simulink model "inc_enc_v26"  (R2022b)
settings: Solver=FixedStepDiscrete  StartTime=0.0  StopTime=SimulationsDauer  RelTol=1e-3
values from neighbouring files (symbols this model uses):
  f_ISR = 40e3    (= 40000)    [Init_IncreEncoder_v26.m]
  IncPerTurn = 2500    [Init_IncreEncoder_v26.m]
  inital_zero_speed_timeout = speed_timeout_in_s*f_fpga    (= 5000)    [Init_IncreEncoder_v26.m]
  n_max = 6000    [Init_IncreEncoder_v26.m]
  Offset_Position_elec = 42    [Init_IncreEncoder_v26.m]
  Offset_Position_mech = 753    [Init_IncreEncoder_v26.m]
  OmegaPerOverSampl = 1500*((2*pi)/60)    (= 157.079632679)    [Init_IncreEncoder_v26.m]
  Periode = abs(1/Striche_pro_Sekunde)    [Init_IncreEncoder_v26.m]
  Phase_Delay_A = Periode/8    [Init_IncreEncoder_v26.m]
  Phase_Delay_B = -Periode/8    [Init_IncreEncoder_v26.m]
  PolePair = 10    [Init_IncreEncoder_v26.m]
  QuadratureFactor = 4    [Init_IncreEncoder_v26.m]
  reciprocal_iterations = 3    [Init_IncreEncoder_v26.m]
  T_fpga = 1/f_fpga    (= 1e-08)    [Init_IncreEncoder_v26.m]
  T_mech = 1e-08    [Init_IncreEncoder_v26.m]
undefined symbols (not defined in the file or in its folder): CW_CCW_Switch, d_axis_hit_CompareValue, DiscIntNeverNeededParam
libraries: hdlsllib x4, dspsrcs4 x3, dspswit3 x2, spsEdgeDetectorLib x2, simulink_extras x1
(part 1 of 2)
settings Model: DataTypeOverride=Off  Creator=Wendel_ELSYS  LastModifiedBy=Admin
settings SolverCC: ConcurrentTasks=on  AlgebraicLoopSolver=TrustRegion  MinimalZcImpactIntegration=on
settings DataIOCC: LimitDataPoints=on  SaveFormat=Array
settings OptimizationCC: BlockReduction=off  ConditionallyExecuteInputs=off  DefaultParameterBehavior=Inlined  InheritOutputTypeSmallerThanSingle=on  LifeSpan=inf
settings DebuggingCC: ReadBeforeWriteMsg=DisableAll  WriteAfterWriteMsg=DisableAll  WriteAfterReadMsg=DisableAll  AlgebraicLoopMsg=error  SingleTaskRateTransMsg=error  ParameterOverflowMsg=none  UnconnectedInputMsg=warning  UnconnectedOutputMsg=warning  UnconnectedLineMsg=warning  SFUnexpectedBacktrackingDiag=warning  SFNoUnconditionalDefaultTransitionDiag=warning  SFExecutionAtInitializationDiag=none  SFMachineParentedDataDiag=warning  ArithmeticOperatorsInVariantConditions=warning
settings HardwareCC: ProdBitPerPointer=32  ProdBitPerSizeT=32  ProdBitPerPtrDiffT=32  ProdLargestAtomicFloat=None  ProdIntDivRoundTo=Undefined  ProdEndianess=Unspecified  ProdWordSize=32  ProdHWDeviceType=ASIC/FPGA->ASIC/FPGA  ProdEqTarget=off
settings ModelReferenceCC: UpdateModelReferenceTargets=IfOutOfDate  EnableRefExpFcnMdlSchedulingChecks=on  PropagateSignalLabelsOutOfModel=off
settings SFSimCC: SFSimEcho=off  SimUseLocalCustomCode=off  CustomCodeUndefinedFunction=UseInterfaceOnly
settings RTWCC: RTWUseLocalCustomCode=off  DLArmComputeVersion=19.05
settings CodeAppCC: StateflowObjectComments=on
settings GRTTargetCC: TargetLangStandard=C89/C90 (ANSI)
settings ConfigComp: CovMetricSettings=dw  CovSaveCumulativeToWorkspaceVar=on  CovSaveSingleToWorkspaceVar=on  CovExternalEMLEnable=off
settings SimscapeCC: SimscapeNormalizeSystem=off

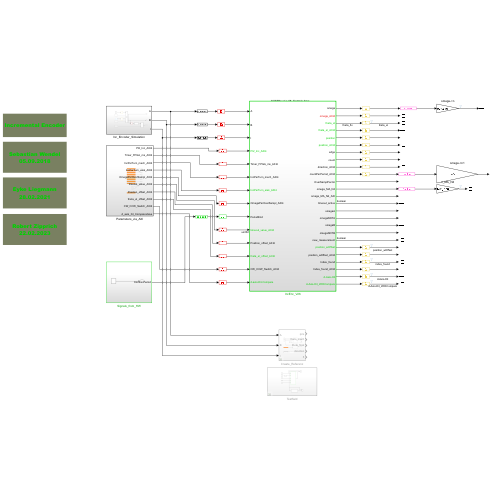
[thumbnail: Simulink's stored preview of the top-level diagram]
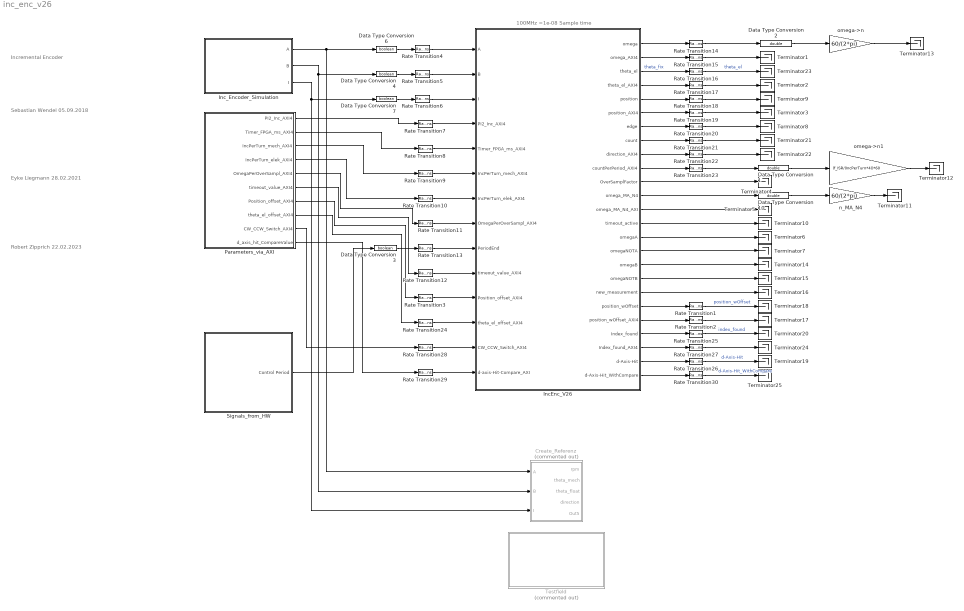
== system inc_enc_v26 ==
  note: 100MHz =1e-08 Sample time
  note: Sebastian Wendel
      | 05.09.2018
  note: Incremental Encoder
  note: Eyke Liegmann
      | 28.02.2021
  note: Robert Zipprich
      | 22.02.2023
  Create_Referenz : Subsystem  Commented=on
  Data Type Conversion1 : DataTypeConversion  OutDataTypeStr=double  SaturateOnIntegerOverflow=off  RndMeth=Floor
  Data Type Conversion10 : DataTypeConversion  OutDataTypeStr=double  SaturateOnIntegerOverflow=off  RndMeth=Floor
  Data Type Conversion2 : DataTypeConversion  OutDataTypeStr=double  SaturateOnIntegerOverflow=off  RndMeth=Floor
  Data Type Conversion{3..4,6..7} (4 alike) : DataTypeConversion  OutDataTypeStr=boolean  SaturateOnIntegerOverflow=off  RndMeth=Floor
  IncEnc_V26 : Subsystem  TreatAsAtomicUnit=on
  Inc_Encoder_Simulation : Subsystem
  Parameters_via_AXI : Subsystem
  Rate Transition{1..2,14..23,25..27,30} (16 alike) : RateTransition  Deterministic=off  OutPortSampleTime=T_mech
  Rate Transition{3..13,24,28..29} (14 alike) : RateTransition  Deterministic=off  OutPortSampleTime=T_fpga
  Signals_from_HW : Subsystem
  Terminator{1..25} (25 alike) : Terminator
  Testfield : Subsystem  Commented=on
  n_MA_N4 : Gain  Gain=60/(2*pi)  OutDataTypeStr=double
  omega->n : Gain  Gain=60/(2*pi)  OutDataTypeStr=double
  omega->n1 : Gain  Gain=(f_ISR/(IncPerTurn*4))*60  OutDataTypeStr=double
  wires:
  Data Type Conversion6/1 -> Rate Transition4/1
  Data Type Conversion4/1 -> Rate Transition5/1
  Data Type Conversion7/1 -> Rate Transition6/1
  IncEnc_V26/1(omega) -> Rate Transition14/1
  IncEnc_V26/9(direction_AXI4) -> Rate Transition22/1
  IncEnc_V26/7(edge) -> Rate Transition20/1
  IncEnc_V26/8(count) -> Rate Transition21/1
  IncEnc_V26/3(theta_el) -> Rate Transition16/1  "theta_fix"
  IncEnc_V26/5(position) -> Rate Transition18/1
  IncEnc_V26/4(theta_el_AXI4) -> Rate Transition17/1
  IncEnc_V26/2(omega_AXI4) -> Rate Transition15/1
  omega->n/1 -> Terminator13/1
  Data Type Conversion2/1 -> omega->n/1
  Data Type Conversion1/1 -> omega->n1/1
  IncEnc_V26/10(countPerPeriod_AXI4) -> Rate Transition23/1
  Data Type Conversion3/1 -> Rate Transition13/1
  IncEnc_V26/6(position_AXI4) -> Rate Transition19/1
  Rate Transition4/1 -> IncEnc_V26/1(A)
  Rate Transition5/1 -> IncEnc_V26/2(B)
  Rate Transition6/1 -> IncEnc_V26/3(I)
  Rate Transition7/1 -> IncEnc_V26/4(PI2_Inc_AXI4)
  Rate Transition8/1 -> IncEnc_V26/5(Timer_FPGA_ms_AXI4)
  Rate Transition9/1 -> IncEnc_V26/6(IncPerTurn_mech_AXI4)
  Rate Transition10/1 -> IncEnc_V26/7(IncPerTurn_elek_AXI4)
  Rate Transition11/1 -> IncEnc_V26/8(OmegaPerOverSampl_AXI4)
  Rate Transition13/1 -> IncEnc_V26/9(PeriodEnd)
  Rate Transition14/1 -> Data Type Conversion2/1
  Rate Transition15/1 -> Terminator1/1
  Rate Transition17/1 -> Terminator2/1
  Rate Transition19/1 -> Terminator3/1
  Rate Transition23/1 -> Data Type Conversion1/1
  IncEnc_V26/11(OverSamplFactor) -> Terminator4/1
  IncEnc_V26/12(omega_MA_N4) -> Data Type Conversion10/1
  IncEnc_V26/13(omega_MA_N4_AXI) -> Terminator5/1
  Data Type Conversion10/1 -> n_MA_N4/1
  Rate Transition12/1 -> IncEnc_V26/10(timeout_value_AXI4)
  IncEnc_V26/14(timeout_active) -> Terminator10/1
  Rate Transition20/1 -> Terminator8/1
  Rate Transition18/1 -> Terminator9/1
  n_MA_N4/1 -> Terminator11/1
  omega->n1/1 -> Terminator12/1
  IncEnc_V26/15(omegaA) -> Terminator6/1
  IncEnc_V26/18(omegaNOTB) -> Terminator15/1
  IncEnc_V26/17(omegaB) -> Terminator14/1
  IncEnc_V26/16(omegaNOTA) -> Terminator7/1
  IncEnc_V26/19(new_measurement) -> Terminator16/1
  Parameters_via_AXI/1(PI2_Inc_AXI4) -> Rate Transition7/1
  Parameters_via_AXI/2(Timer_FPGA_ms_AXI4) -> Rate Transition8/1
  Parameters_via_AXI/3(IncPerTurn_mech_AXI4) -> Rate Transition9/1
  Parameters_via_AXI/4(IncPerTurn_elek_AXI4) -> Rate Transition10/1
  Parameters_via_AXI/5(OmegaPerOverSampl_AXI4) -> Rate Transition11/1
  Parameters_via_AXI/6(timeout_value_AXI4) -> Rate Transition12/1
  Inc_Encoder_Simulation/2(B) -> Create_Referenz/2(B), Data Type Conversion4/1
  Inc_Encoder_Simulation/3(I) -> Create_Referenz/3(I), Data Type Conversion7/1
  Inc_Encoder_Simulation/1(A) -> Data Type Conversion6/1, Create_Referenz/1(A)
  Signals_from_HW/1(Control Period) -> Data Type Conversion3/1
  Rate Transition1/1 -> Terminator18/1  "position_wOffset"
  Rate Transition2/1 -> Terminator17/1
  IncEnc_V26/21(position_wOffset_AXI4) -> Rate Transition2/1
  IncEnc_V26/20(position_wOffset) -> Rate Transition1/1
  Rate Transition3/1 -> IncEnc_V26/11(Position_offset_AXI4)
  Parameters_via_AXI/7(Position_offset_AXI4) -> Rate Transition3/1
  Rate Transition24/1 -> IncEnc_V26/12(theta_el_offset_AXI4)
  Parameters_via_AXI/8(theta_el_offset_AXI4) -> Rate Transition24/1
  IncEnc_V26/22(Index_found) -> Rate Transition25/1
  Rate Transition25/1 -> Terminator20/1  "index_found"
  Rate Transition26/1 -> Terminator19/1  "d-Axis-Hit"
  IncEnc_V26/24(d-Axis-Hit) -> Rate Transition26/1
  Rate Transition22/1 -> Terminator22/1
  Rate Transition21/1 -> Terminator21/1
  Rate Transition16/1 -> Terminator23/1  "theta_el"
  Rate Transition27/1 -> Terminator24/1
  IncEnc_V26/23(Index_found_AXI4) -> Rate Transition27/1
  Rate Transition28/1 -> IncEnc_V26/13(CW_CCW_Switch_AXI4)
  Parameters_via_AXI/9(CW_CCW_Switch_AXI4) -> Rate Transition28/1
  Rate Transition29/1 -> IncEnc_V26/14(d-axis-Hit-Compare_AXI)
  Parameters_via_AXI/10(d_axis_hit_CompareValue) -> Rate Transition29/1
  IncEnc_V26/25(d-Axis-Hit_WithCompare) -> Rate Transition30/1
  Rate Transition30/1 -> Terminator25/1  "d-Axis-Hit_WithCompare"

== system inc_enc_v26/Create_Referenz ==
  note: Überprüfen der Ausgabe:
      | (1/((Wert in Periodfelt von Counter)*Inkremente))*60
      | z.B. (1/((2.5*0.000001)*5000))*60
  A : Inport
  B : Inport  Port=2
  I : Inport  Port=3
  HardwareTimer_FPGA_in_ms*InCrements1 : Constant  Value=T_mech*IncPerTurn  OutDataTypeStr=double  SampleTime=T_mech
  IncrementalEncoder_Floating : Subsystem  Commented=on
  "daQuadraturEncoder " : Gain  Commented=on  Gain=4
  n_aus_theta : Subsystem  Commented=on  TreatAsAtomicUnit=on
  poles : Constant  Value=PolePair  OutDataTypeStr=uint8  SampleTime=T_mech
  rpm : Outport
  theta_mech : Outport  Port=2
  theta_float : Outport  Port=3
  direction : Outport  Port=4
  Out5 : Outport  Port=5
  wires:
  n_aus_theta/1(rpm) -> "daQuadraturEncoder "/1
  A/1 -> IncrementalEncoder_Floating/1(A), n_aus_theta/1(count)
  B/1 -> IncrementalEncoder_Floating/2(B)
  IncrementalEncoder_Floating/3(theta_elec) -> theta_float/1  "theta_float"
  poles/1 -> IncrementalEncoder_Floating/4(poles)
  I/1 -> IncrementalEncoder_Floating/3(I)
  HardwareTimer_FPGA_in_ms*InCrements1/1 -> n_aus_theta/2(T)
  IncrementalEncoder_Floating/4(direction) -> direction/1
  IncrementalEncoder_Floating/1(rpm) -> rpm/1
  "daQuadraturEncoder "/1 -> Out5/1
  IncrementalEncoder_Floating/2(theta_mech) -> theta_mech/1

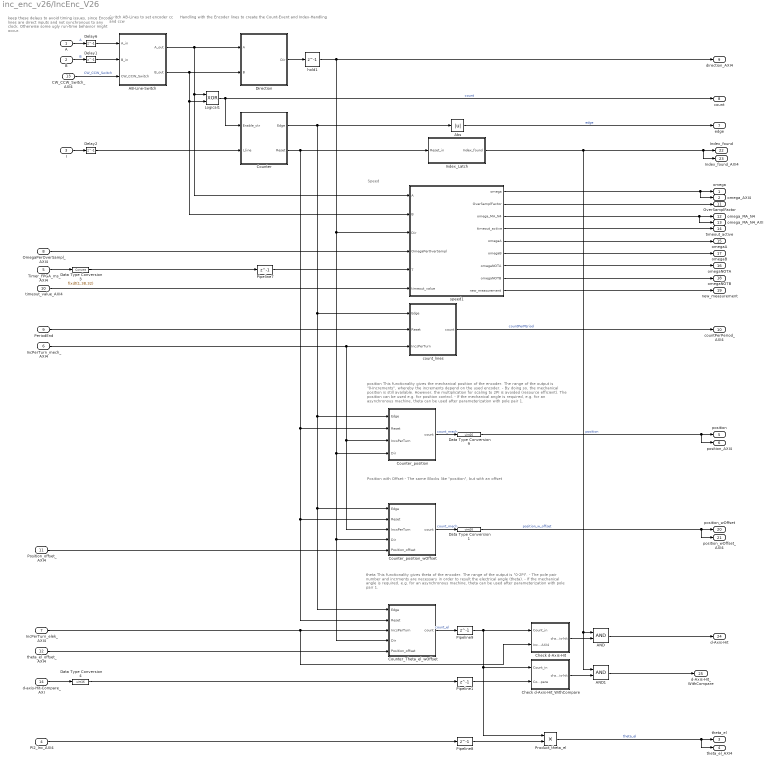
== system inc_enc_v26/IncEnc_V26 ==
  note: Switch AB-Lines to set
      | encoder cc and ccw
  note: Handling with the Encoder lines to create the Count-Event and Index-Handling
  note: Speed
  note: position
      | This functionality gives the mechanical position of the encoder. The range of the output is "0-Increments", whereby the increments depend on the used encoder.
      | - By doing so, the mechanical position is still available. However, the multiplication for scaling to 2PI is avoided (resource efficient). The position can be used e.g. for position control.
      | - If the mechanical angle is required, e.g. for an asynchronous machine, theta can be used after parameterization with pole pair 1.
  note: theta
      | This functionality gives theta of the encoder. The range of the output is "0-2PI".
      | - The pole pair number and incrments are necessary in order to result the electrical angle (theta).
      | - If the mechanical angle is required, e.g. for an asynchronous machine, theta can be used after parameterization with pole pair 1.
  note: keep these delays to avoid timing issues,
      | since Encoder lines are direct inputs and
      | not synchronous to any clock.
      | Otherwise some ugly run-time
      | behavior might occur.
  note: Position with Offset
      | - The same Blocks like "position", but with an offset
  A : Inport
  B : Inport  Port=2
  I : Inport  Port=3
  PI2_Inc_AXI4 : Inport  Port=4
  Timer_FPGA_ms_AXI4 : Inport  Port=5
  IncPerTurn_mech_AXI4 : Inport  Port=6
  IncPerTurn_elek_AXI4 : Inport  Port=7
  OmegaPerOverSampl_AXI4 : Inport  Port=8
  PeriodEnd : Inport  Port=9
  timeout_value_AXI4 : Inport  Port=10  OutDataTypeStr=uint32
  Position_offset_AXI4 : Inport  Port=11
  theta_el_offset_AXI4 : Inport  Port=12
  CW_CCW_Switch_AXI4 : Inport  Port=13
  d-axis-Hit-Compare_AXI : Inport  Port=14
  AB-Line-Switch : Subsystem
  AND : Logic  AllPortsSameDT=off  OutDataTypeStr=boolean
  AND1 : Logic  AllPortsSameDT=off  OutDataTypeStr=boolean
  Abs : Abs  OutDataTypeStr=fixdt(0,1,0)  RndMeth=Simplest  SaturateOnIntegerOverflow=off
  Check d-Axis-Hit : Subsystem
  Check d-Axis-Hit_WithCompare : Subsystem
  Counter : Subsystem  TreatAsAtomicUnit=on
  Counter_Theta_el_wOffset : Subsystem  TreatAsAtomicUnit=on
  Counter_position : Subsystem  TreatAsAtomicUnit=on
  Counter_position_wOffset : Subsystem  TreatAsAtomicUnit=on
  Data Type Conversion1 : DataTypeConversion  OutDataTypeStr=uint16  SaturateOnIntegerOverflow=off  RndMeth=Floor
  Data Type Conversion3 : DataTypeConversion  OutDataTypeStr=fixdt(1,38,32)  SaturateOnIntegerOverflow=off  RndMeth=Floor
  Data Type Conversion4 : DataTypeConversion  OutDataTypeStr=uint16  SaturateOnIntegerOverflow=off  RndMeth=Floor
  Data Type Conversion9 : DataTypeConversion  OutDataTypeStr=uint16  SaturateOnIntegerOverflow=off  RndMeth=Floor
  Delay1 : Delay  DelayLength=1  InitialCondition=0
  Delay2 : Delay  DelayLength=1  InitialCondition=0
  Delay6 : Delay  DelayLength=1  InitialCondition=0
  Direction : Subsystem  TreatAsAtomicUnit=on
  Index_Latch : Subsystem
  Logical1 : Logic  Operator=XOR  AllPortsSameDT=off  OutDataTypeStr=boolean
  Pipeline{1,7..9} (4 alike) : Delay  DelayLength=1
  Product_theta_el : Product  OutMin=[0]  OutMax=[2*pi]  OutDataTypeStr=fixdt(1,24,20)
  count_lines : Subsystem  TreatAsAtomicUnit=on
  hold1 : Delay  DelayLength=1
  speed1 : Subsystem
  omega : Outport  VectorParamsAs1DForOutWhenUnconnected=off
  omega_AXI4 : Outport  Port=2  VectorParamsAs1DForOutWhenUnconnected=off
  theta_el : Outport  Port=3  VectorParamsAs1DForOutWhenUnconnected=off
  theta_el_AXI4 : Outport  Port=4  VectorParamsAs1DForOutWhenUnconnected=off
  position : Outport  Port=5  VectorParamsAs1DForOutWhenUnconnected=off
  position_AXI4 : Outport  Port=6  VectorParamsAs1DForOutWhenUnconnected=off
  edge : Outport  Port=7  VectorParamsAs1DForOutWhenUnconnected=off
  count : Outport  Port=8  VectorParamsAs1DForOutWhenUnconnected=off
  direction_AXI4 : Outport  Port=9  VectorParamsAs1DForOutWhenUnconnected=off
  countPerPeriod_AXI4 : Outport  Port=10  VectorParamsAs1DForOutWhenUnconnected=off
  OverSamplFactor : Outport  Port=11  VectorParamsAs1DForOutWhenUnconnected=off
  omega_MA_N4 : Outport  Port=12  VectorParamsAs1DForOutWhenUnconnected=off
  omega_MA_N4_AXI : Outport  Port=13  VectorParamsAs1DForOutWhenUnconnected=off
  timeout_active : Outport  Port=14  OutDataTypeStr=boolean  VectorParamsAs1DForOutWhenUnconnected=off
  omegaA : Outport  Port=15  VectorParamsAs1DForOutWhenUnconnected=off
  omegaNOTA : Outport  Port=16  VectorParamsAs1DForOutWhenUnconnected=off
  omegaB : Outport  Port=17  VectorParamsAs1DForOutWhenUnconnected=off
  omegaNOTB : Outport  Port=18  VectorParamsAs1DForOutWhenUnconnected=off
  new_measurement : Outport  Port=19  OutDataTypeStr=boolean  VectorParamsAs1DForOutWhenUnconnected=off
  position_wOffset : Outport  Port=20  VectorParamsAs1DForOutWhenUnconnected=off
  position_wOffset_AXI4 : Outport  Port=21  VectorParamsAs1DForOutWhenUnconnected=off
  Index_found : Outport  Port=22  VectorParamsAs1DForOutWhenUnconnected=off
  Index_found_AXI4 : Outport  Port=23  VectorParamsAs1DForOutWhenUnconnected=off
  d-Axis-Hit : Outport  Port=24  VectorParamsAs1DForOutWhenUnconnected=off
  d-Axis-Hit_WithCompare : Outport  Port=25  VectorParamsAs1DForOutWhenUnconnected=off
  wires:
  A/1 -> Delay6/1  "A"
  B/1 -> Delay1/1  "B"
  hold1/1 -> direction_AXI4/1, speed1/3(Dir), Counter_position/4(Dir), Counter_Theta_el_wOffset/4(Dir), Counter_position_wOffset/4(Dir)
  Counter_position/1(count) -> Data Type Conversion9/1  "count_mech"
  Data Type Conversion9/1 -> position_AXI4/1, position/1  "position"
  Logical1/1 -> Counter/1(Enable_ctr), count/1  "count"
  Counter_Theta_el_wOffset/1(count) -> Pipeline9/1  "count_el"
  Product_theta_el/1 -> theta_el/1, theta_el_AXI4/1  "theta_el"
  Counter/2(Reset) -> Counter_position/2(Reset), Counter_Theta_el_wOffset/2(Reset), Counter_position_wOffset/2(Reset), Index_Latch/1(Reset_in)
  Counter/1(Edge) -> Counter_position/1(Edge), Counter_Theta_el_wOffset/1(Edge), Counter_position_wOffset/1(Edge), count_lines/1(Edge), Abs/1
  Direction/1(Dir) -> hold1/1
  PeriodEnd/1 -> count_lines/2(Reset)
  count_lines/1(count) -> countPerPeriod_AXI4/1  "countPerPEriod"
  Abs/1 -> edge/1  "edge"
  IncPerTurn_elek_AXI4/1 -> Counter_Theta_el_wOffset/3(IncsPerTurn), Check d-Axis-Hit/2(IncPerTurn_elek_AXI4)
  IncPerTurn_mech_AXI4/1 -> Counter_position/3(IncsPerTurn), Counter_position_wOffset/3(IncsPerTurn), count_lines/3(IncsPerTurn)
  Timer_FPGA_ms_AXI4/1 -> Data Type Conversion3/1
  Data Type Conversion3/1 -> Pipeline7/1
  OmegaPerOverSampl_AXI4/1 -> speed1/4(OmegaPerOverSampl)
  Pipeline7/1 -> speed1/5(T)
  speed1/1(omega) -> omega_AXI4/1, omega/1
  speed1/2(OverSamplFactor) -> OverSamplFactor/1
  speed1/3(omega_MA_N4) -> omega_MA_N4_AXI/1, omega_MA_N4/1
  speed1/4(timeout_active) -> timeout_active/1
  timeout_value_AXI4/1 -> speed1/6(timeout_value)
  speed1/5(omegaA) -> omegaA/1
  speed1/7(omegaNOTA) -> omegaNOTA/1
  speed1/6(omegaB) -> omegaB/1
  speed1/8(omegaNOTB) -> omegaNOTB/1
  speed1/9(new_measurement) -> new_measurement/1
  AB-Line-Switch/1(A_out) -> speed1/1(A), Logical1/1, Direction/1(A)
  AB-Line-Switch/2(B_out) -> speed1/2(B), Logical1/2, Direction/2(B)
  Counter_position_wOffset/1(count) -> Data Type Conversion1/1  "count_mech"
  Data Type Conversion1/1 -> position_wOffset_AXI4/1, position_wOffset/1  "position_w_offset"
  Position_offset_AXI4/1 -> Counter_position_wOffset/5(Position_offset)
  I/1 -> Delay2/1
  Delay2/1 -> Counter/2(I_line)
  theta_el_offset_AXI4/1 -> Counter_Theta_el_wOffset/5(Position_offset)
  Pipeline9/1 -> Check d-Axis-Hit_WithCompare/1(Count_in), Product_theta_el/1, Check d-Axis-Hit/1(Count_in)
  Pipeline8/1 -> Product_theta_el/2
  Check d-Axis-Hit/1(d-axis-hit) -> AND/2
  AND/1 -> d-Axis-Hit/1
  Index_Latch/1(Index_found) -> Index_found_AXI4/1, Index_found/1, AND1/1, AND/1
  Delay6/1 -> AB-Line-Switch/1(A_in)
  Delay1/1 -> AB-Line-Switch/2(B_in)
  CW_CCW_Switch_AXI4/1 -> AB-Line-Switch/3(CW_CCW_Switch)  "CW_CCW_Switch"
  Check d-Axis-Hit_WithCompare/1(d-axis-hit) -> AND1/2
  AND1/1 -> d-Axis-Hit_WithCompare/1
  d-axis-Hit-Compare_AXI/1 -> Data Type Conversion4/1
  Pipeline1/1 -> Check d-Axis-Hit_WithCompare/2(Counter_Compare)
  PI2_Inc_AXI4/1 -> Pipeline8/1
  Data Type Conversion4/1 -> Pipeline1/1

== system inc_enc_v26/Inc_Encoder_Simulation ==
  Logical Operator1 : Logic  Operator=XOR  AllPortsSameDT=off  OutDataTypeStr=boolean
  Manual Switch : ManualSwitch
  Manual Switch1 : ManualSwitch
  Manual Switch2 : ManualSwitch
  Pulse Generator1 0.1 : DiscretePulseGenerator  PulseType=Time based  Period=Periode  PulseWidth=50  PhaseDelay=Phase_Delay_B  SampleTime=T_mech  VectorParams1D=off
  Pulse Generator2 : DiscretePulseGenerator  PulseType=Time based  Period=Periode  PulseWidth=50  PhaseDelay=Phase_Delay_A  SampleTime=T_mech  VectorParams1D=off
  Rate Transition : RateTransition  Deterministic=off  OutPortSampleTime=T_mech
  Rate Transition2 : RateTransition  Deterministic=off  OutPortSampleTime=T_mech
  Signal From Workspace : dspsrcs4/Signal From Workspace  Commented=on  X=A_ila  Ts=T_mech  nsamps=1  OutputAfterFinalValue=Setting to zero  ignoreOrWarnInputAndFrameLengths=off  OutputFrames=off
  Signal From Workspace1 : dspsrcs4/Signal From Workspace  Commented=on  X=B_ila  Ts=T_mech  nsamps=1  OutputAfterFinalValue=Setting to zero  ignoreOrWarnInputAndFrameLengths=off  OutputFrames=off
  Signal From Workspace2 : dspsrcs4/Signal From Workspace  Commented=on  X=I_ila  Ts=T_mech  nsamps=1  OutputAfterFinalValue=Setting to zero  ignoreOrWarnInputAndFrameLengths=off  OutputFrames=off
  Simulate_I_Line : dspswit3/Counter  Direction=Up  CountEvent=Either edge  CounterSize=User defined  MaxCount=IncPerTurn*4  InitialCount=123  Output=Hit  HitValue=IncPerTurn*4  ResetInput=off  SamplesPerFrame=1  Ts=1  CntDtype=double  HitDtype=Boolean
  A : Outport
  B : Outport  Port=2
  I : Outport  Port=3
  wires:
  Pulse Generator2/1 -> Rate Transition/1  "A"
  Signal From Workspace1/1 -> Manual Switch1/2
  Logical Operator1/1 -> Simulate_I_Line/1
  Manual Switch1/1 -> B/1, Logical Operator1/2
  Signal From Workspace/1 -> Manual Switch/2
  Manual Switch/1 -> A/1, Logical Operator1/1
  Pulse Generator1 0.1/1 -> Rate Transition2/1  "B"
  Rate Transition/1 -> Manual Switch/1
  Rate Transition2/1 -> Manual Switch1/1
  Signal From Workspace2/1 -> Manual Switch2/2
  Simulate_I_Line/1 -> Manual Switch2/1
  Manual Switch2/1 -> I/1  "I"

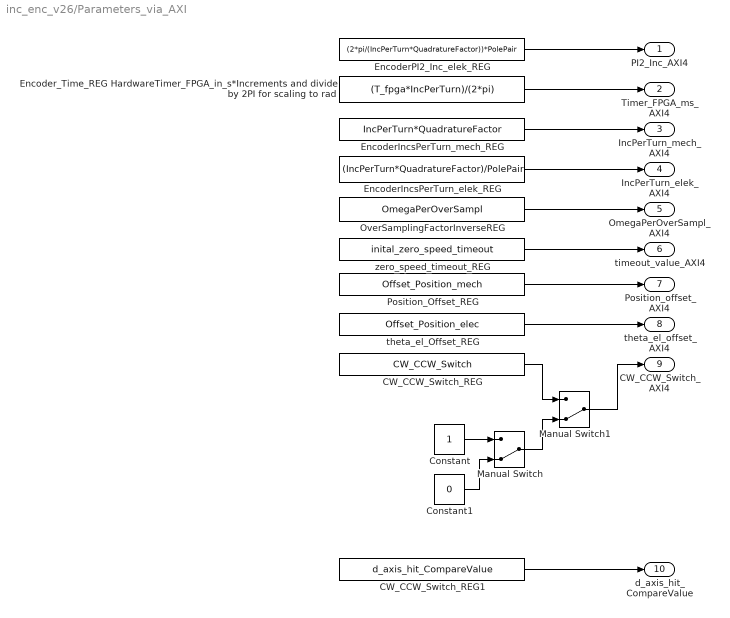
== system inc_enc_v26/Parameters_via_AXI ==
  CW_CCW_Switch_REG : Constant  Value=CW_CCW_Switch  OutDataTypeStr=boolean  SampleTime=T_mech
  CW_CCW_Switch_REG1 : Constant  Value=d_axis_hit_CompareValue  OutDataTypeStr=uint32  SampleTime=T_mech
  Constant : Constant  OutDataTypeStr=boolean
  Constant1 : Constant  Value=0  OutDataTypeStr=boolean
  "EncoderIncsPerTurn_elek_REG " : Constant  Value=(IncPerTurn*QuadratureFactor)/PolePair  OutDataTypeStr=fixdt(0,16,0)  SampleTime=T_mech
  EncoderIncsPerTurn_mech_REG : Constant  Value=IncPerTurn*QuadratureFactor  OutDataTypeStr=fixdt(0,16,0)  SampleTime=T_mech
  EncoderPI2_Inc_elek_REG : Constant  Value=(2*pi/(IncPerTurn*QuadratureFactor))*PolePair  OutDataTypeStr=fixdt(0,24,24)  SampleTime=T_mech
  Encoder_Time_REG HardwareTimer_FPGA_in_s*Increments and divide by 2PI for scaling to rad : Constant  Value=(T_fpga*IncPerTurn)/(2*pi)  OutDataTypeStr=fixdt(0,32,32)  SampleTime=T_mech
  Manual Switch : ManualSwitch  CurrentSetting=0
  Manual Switch1 : ManualSwitch  CurrentSetting=0
  OverSamplingFactorInverseREG : Constant  Value=OmegaPerOverSampl  OutDataTypeStr=fixdt(1,24,11)  SampleTime=T_mech
  Position_Offset_REG : Constant  Value=Offset_Position_mech  OutDataTypeStr=fixdt(0,16,0)  SampleTime=T_mech
  theta_el_Offset_REG : Constant  Value=Offset_Position_elec  OutDataTypeStr=fixdt(0,16,0)  SampleTime=T_mech
  zero_speed_timeout_REG : Constant  Value=inital_zero_speed_timeout  OutDataTypeStr=uint32  SampleTime=T_mech
  PI2_Inc_AXI4 : Outport
  Timer_FPGA_ms_AXI4 : Outport  Port=2
  IncPerTurn_mech_AXI4 : Outport  Port=3
  IncPerTurn_elek_AXI4 : Outport  Port=4
  OmegaPerOverSampl_AXI4 : Outport  Port=5
  timeout_value_AXI4 : Outport  Port=6
  Position_offset_AXI4 : Outport  Port=7
  theta_el_offset_AXI4 : Outport  Port=8
  CW_CCW_Switch_AXI4 : Outport  Port=9
  d_axis_hit_CompareValue : Outport  Port=10
  wires:
  "EncoderIncsPerTurn_elek_REG "/1 -> IncPerTurn_elek_AXI4/1
  Encoder_Time_REG HardwareTimer_FPGA_in_s*Increments and divide by 2PI for scaling to rad/1 -> Timer_FPGA_ms_AXI4/1
  zero_speed_timeout_REG/1 -> timeout_value_AXI4/1
  OverSamplingFactorInverseREG/1 -> OmegaPerOverSampl_AXI4/1
  EncoderPI2_Inc_elek_REG/1 -> PI2_Inc_AXI4/1
  EncoderIncsPerTurn_mech_REG/1 -> IncPerTurn_mech_AXI4/1
  Position_Offset_REG/1 -> Position_offset_AXI4/1
  theta_el_Offset_REG/1 -> theta_el_offset_AXI4/1
  Constant/1 -> Manual Switch/1
  Constant1/1 -> Manual Switch/2
  CW_CCW_Switch_REG/1 -> Manual Switch1/1
  Manual Switch/1 -> Manual Switch1/2
  Manual Switch1/1 -> CW_CCW_Switch_AXI4/1
  CW_CCW_Switch_REG1/1 -> d_axis_hit_CompareValue/1

== system inc_enc_v26/Signals_from_HW ==
  uCTakt : DiscretePulseGenerator  PulseType=Time based  Period=1/f_ISR  PulseWidth=f_ISR*T_fpga *100  SampleTime=T_mech  VectorParams1D=off
  Control Period : Outport
  wires:
  uCTakt/1 -> Control Period/1  "Control Period"

== system inc_enc_v26/Testfield ==
  Cast To Boolean1 : DataTypeConversion  OutDataTypeStr=boolean  SaturateOnIntegerOverflow=off  RndMeth=Floor
  Constant1 : Constant  Value=256*4
  Constant2 : Constant
  Constant3 : Constant  Value=512
  Counter_position_wOffset : Subsystem  TreatAsAtomicUnit=on
  Index_Latch : Subsystem
  Pulse Generator : DiscretePulseGenerator  Period=10  SampleTime=1/10e3
  Pulse Generator1 : DiscretePulseGenerator  Period=100000  PhaseDelay=42505  SampleTime=1/10e3
  Scope : Scope  NumInputPorts=3
  Scope1 : Scope  NumInputPorts=2
  wires:
  Constant1/1 -> Counter_position_wOffset/3(IncsPerTurn)
  Pulse Generator/1 -> Counter_position_wOffset/1(Edge), Scope/1
  Constant3/1 -> Counter_position_wOffset/5(Position_offset)
  Constant2/1 -> Counter_position_wOffset/4(Dir)
  Cast To Boolean1/1 -> Scope/2, Scope1/1, Index_Latch/1(Reset_in), Counter_position_wOffset/2(Reset)
  Pulse Generator1/1 -> Cast To Boolean1/1
  Counter_position_wOffset/1(count) -> Scope/3  "count_mech"
  Index_Latch/1(Index_found) -> Scope1/2

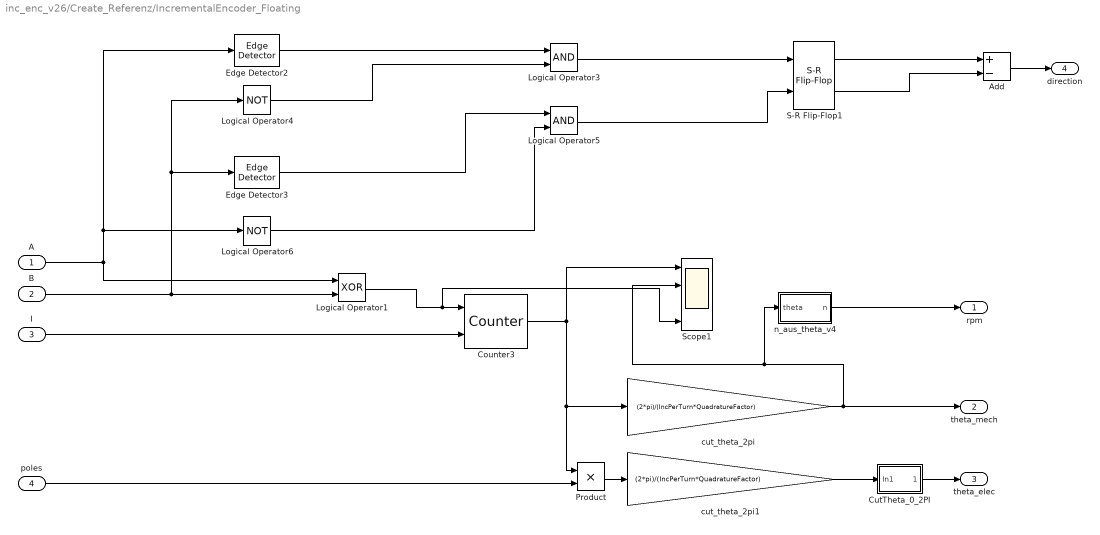
== system inc_enc_v26/Create_Referenz/IncrementalEncoder_Floating ==
  A : Inport
  B : Inport  Port=2
  I : Inport  Port=3
  poles : Inport  Port=4
  Add : Sum  Inputs=+-  OutDataTypeStr=fixdt(1,16,0)
  Counter3 : dspswit3/Counter  Direction=Up  CountEvent=Either edge  CounterSize=User defined  MaxCount=IncPerTurn*4  InitialCount=0  Output=Count  HitValue=32  ResetInput=on  SamplesPerFrame=1  Ts=1  CntDtype=double  HitDtype=Logical
  CutTheta_0_2PI : Subsystem
  Edge Detector2 : spsEdgeDetectorLib/Edge Detector  model=Rising  ic=0  Ts=-1
  Edge Detector3 : spsEdgeDetectorLib/Edge Detector  model=Rising  ic=0  Ts=-1
  Logical Operator1 : Logic  Operator=XOR  AllPortsSameDT=off  OutDataTypeStr=boolean
  Logical Operator3 : Logic  AllPortsSameDT=off  OutDataTypeStr=boolean
  Logical Operator4 : Logic  Operator=NOT  AllPortsSameDT=off  OutDataTypeStr=boolean
  Logical Operator5 : Logic  AllPortsSameDT=off  OutDataTypeStr=boolean
  Logical Operator6 : Logic  Operator=NOT  AllPortsSameDT=off  OutDataTypeStr=boolean
  Product : Product
  S-R Flip-Flop1 : simulink_extras/Flip Flops/S-R Flip-Flop  initial_condition=0
  Scope1 : Scope  NumInputPorts=4
  cut_theta_2pi : Gain  Gain=(2*pi)/(IncPerTurn*QuadratureFactor)
  cut_theta_2pi1 : Gain  Gain=(2*pi)/(IncPerTurn*QuadratureFactor)
  n_aus_theta_v4 : Subsystem
  rpm : Outport  VectorParamsAs1DForOutWhenUnconnected=off
  theta_mech : Outport  Port=2  VectorParamsAs1DForOutWhenUnconnected=off
  theta_elec : Outport  Port=3  VectorParamsAs1DForOutWhenUnconnected=off
  direction : Outport  Port=4  VectorParamsAs1DForOutWhenUnconnected=off
  wires:
  I/1 -> Counter3/2
  Counter3/1 -> Product/1, cut_theta_2pi/1, Scope1/1
  n_aus_theta_v4/1(n) -> rpm/1
  Logical Operator1/1 -> Scope1/4, Counter3/1
  cut_theta_2pi/1 -> Scope1/2, n_aus_theta_v4/1(theta), theta_mech/1
  Product/1 -> cut_theta_2pi1/1
  poles/1 -> Product/2
  cut_theta_2pi1/1 -> CutTheta_0_2PI/1(In1)
  CutTheta_0_2PI/1(Out1) -> theta_elec/1
  Edge Detector2/1 -> Logical Operator3/1
  Logical Operator4/1 -> Logical Operator3/2
  Logical Operator3/1 -> S-R Flip-Flop1/1
  Edge Detector3/1 -> Logical Operator5/1
  Logical Operator6/1 -> Logical Operator5/2
  Logical Operator5/1 -> S-R Flip-Flop1/2
  S-R Flip-Flop1/1 -> Add/1
  S-R Flip-Flop1/2 -> Add/2
  A/1 -> Logical Operator6/1, Edge Detector2/1, Logical Operator1/1
  B/1 -> Edge Detector3/1, Logical Operator4/1, Logical Operator1/2
  Add/1 -> direction/1

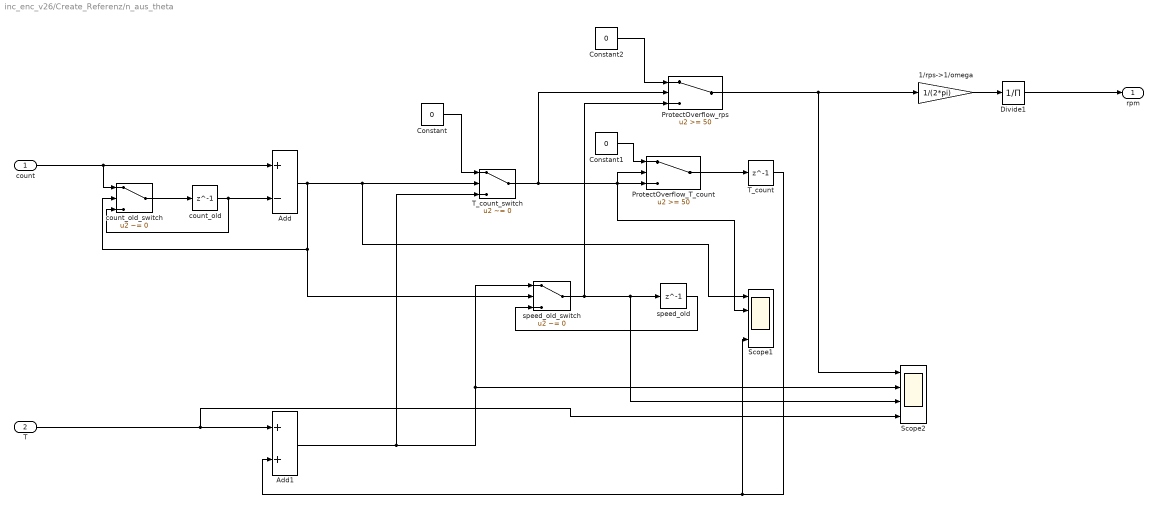
== system inc_enc_v26/Create_Referenz/n_aus_theta ==
  count : Inport
  T : Inport  Port=2
  1/rps->1/omega : Gain  Gain=1/(2*pi)  OutDataTypeStr=double
  Add : Sum  Inputs=+-
  Add1 : Sum
  Constant : Constant  Value=0  OutDataTypeStr=double  SampleTime=-1
  Constant1 : Constant  Value=0  OutDataTypeStr=double  SampleTime=-1
  Constant2 : Constant  Value=0  OutDataTypeStr=double  SampleTime=-1
  Divide1 : Product  Inputs=/
  ProtectOverflow_T_count : Switch  Threshold=50  SaturateOnIntegerOverflow=off  InputSameDT=off
  ProtectOverflow_rps : Switch  Threshold=50  OutDataTypeStr=double  SaturateOnIntegerOverflow=off  InputSameDT=off
  Scope1 : Scope  NumInputPorts=4
  Scope2 : Scope  NumInputPorts=4
  T_count : Delay  DelayLength=1
  T_count_switch : Switch  Criteria=u2 ~= 0  SaturateOnIntegerOverflow=off  InputSameDT=off
  count_old : Delay  DelayLength=1
  count_old_switch : Switch  Criteria=u2 ~= 0  SaturateOnIntegerOverflow=off  InputSameDT=off
  speed_old : Delay  DelayLength=1
  speed_old_switch : Switch  Criteria=u2 ~= 0  SaturateOnIntegerOverflow=off  InputSameDT=off
  rpm : Outport  VectorParamsAs1DForOutWhenUnconnected=off
  wires:
  count_old_switch/1 -> count_old/1
  count_old/1 -> count_old_switch/3, Add/2
  Constant/1 -> T_count_switch/1
  Add/1 -> speed_old_switch/2, count_old_switch/2, Scope1/1, T_count_switch/2
  Constant1/1 -> ProtectOverflow_T_count/1
  ProtectOverflow_rps/1 -> 1/rps->1/omega/1, Scope2/1
  Constant2/1 -> ProtectOverflow_rps/1
  speed_old_switch/1 -> ProtectOverflow_rps/3, Scope2/3, speed_old/1
  speed_old/1 -> speed_old_switch/3
  T/1 -> Scope2/4, Add1/1
  ProtectOverflow_T_count/1 -> T_count/1
  T_count/1 -> Scope1/4, Add1/2
  Add1/1 -> Scope2/2, speed_old_switch/1, T_count_switch/3
  count/1 -> Add/1, count_old_switch/1
  T_count_switch/1 -> ProtectOverflow_rps/2, Scope1/2, ProtectOverflow_T_count/2, ProtectOverflow_T_count/3
  1/rps->1/omega/1 -> Divide1/1
  Divide1/1 -> rpm/1

== system inc_enc_v26/IncEnc_V26/AB-Line-Switch ==
  A_in : Inport
  B_in : Inport  Port=2
  CW_CCW_Switch : Inport  Port=3
  Switch : Switch  Criteria=u2 > Threshold  SaturateOnIntegerOverflow=off  InputSameDT=off
  Switch1 : Switch  Criteria=u2 > Threshold  SaturateOnIntegerOverflow=off  InputSameDT=off
  A_out : Outport
  B_out : Outport  Port=2
  wires:
  Switch/1 -> A_out/1
  Switch1/1 -> B_out/1
  B_in/1 -> Switch/1, Switch1/3
  A_in/1 -> Switch1/1, Switch/3
  CW_CCW_Switch/1 -> Switch1/2, Switch/2

== system inc_enc_v26/IncEnc_V26/Check d-Axis-Hit ==
  Count_in : Inport
  IncPerTurn_elek_AXI4 : Inport  Port=2
  Constant : Constant  Value=0  OutDataTypeStr=Inherit: Inherit via back propagation  SampleTime=T_fpga
  Equal : RelationalOperator  Operator===  OutDataTypeStr=boolean  RndMeth=Simplest  InputSameDT=off
  Equal1 : RelationalOperator  Operator===  OutDataTypeStr=boolean  RndMeth=Simplest  InputSameDT=off
  OR : Logic  Operator=OR  AllPortsSameDT=off  OutDataTypeStr=boolean
  d-axis-hit : Outport  VectorParamsAs1DForOutWhenUnconnected=off
  wires:
  Count_in/1 -> Equal1/1, Equal/1
  Constant/1 -> Equal/2
  IncPerTurn_elek_AXI4/1 -> Equal1/2
  Equal/1 -> OR/1
  Equal1/1 -> OR/2
  OR/1 -> d-axis-hit/1

== system inc_enc_v26/IncEnc_V26/Check d-Axis-Hit_WithCompare ==
  Count_in : Inport
  Counter_Compare : Inport  Port=2
  Equal : RelationalOperator  Operator===  OutDataTypeStr=boolean  RndMeth=Simplest  InputSameDT=off
  d-axis-hit : Outport  VectorParamsAs1DForOutWhenUnconnected=off
  wires:
  Counter_Compare/1 -> Equal/2
  Count_in/1 -> Equal/1
  Equal/1 -> d-axis-hit/1

== system inc_enc_v26/IncEnc_V26/Counter ==
  note: 1 for one cycle if edge recognized
  note: Reset
  Enable_ctr : Inport
  I_line : Inport  Port=2
  Detec_edge : Sum  Inputs=+-  AccumDataTypeStr=int8  OutDataTypeStr=int8
  Reset_flag : Sum  Inputs=+-  AccumDataTypeStr=uint8  OutDataTypeStr=uint8
  reset_old : Delay  DelayLength=1
  reset_old1 : Delay  DelayLength=1
  reset_old_switch : Switch  Criteria=u2 ~= 0  SaturateOnIntegerOverflow=off  InputSameDT=off
  reset_old_switch1 : Switch  Criteria=u2 ~= 0  SaturateOnIntegerOverflow=off  InputSameDT=off
  Edge : Outport  VectorParamsAs1DForOutWhenUnconnected=off
  Reset : Outport  Port=2  VectorParamsAs1DForOutWhenUnconnected=off
  wires:
  I_line/1 -> Reset_flag/1, reset_old_switch/1
  reset_old_switch/1 -> reset_old/1
  reset_old/1 -> reset_old_switch/3, Reset_flag/2
  Reset_flag/1 -> Reset/1, reset_old_switch/2
  Enable_ctr/1 -> Detec_edge/1, reset_old_switch1/1
  reset_old_switch1/1 -> reset_old1/1
  reset_old1/1 -> reset_old_switch1/3, Detec_edge/2
  Detec_edge/1 -> reset_old_switch1/2, Edge/1  "1 for one cycle if edge recognized"

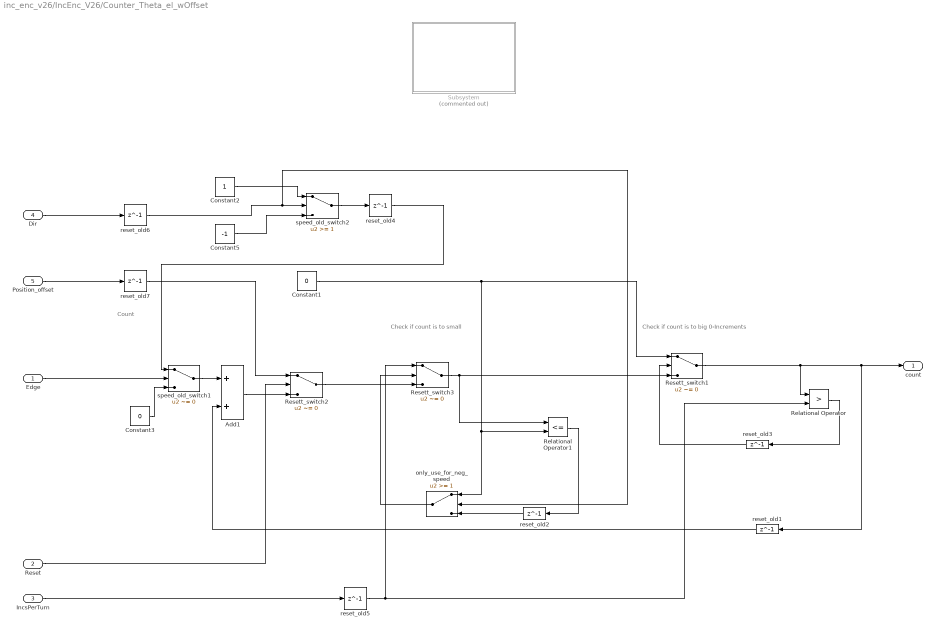
== system inc_enc_v26/IncEnc_V26/Counter_Theta_el_wOffset ==
  note: Check if count is to big 0-Increments
  note: Count
  note: Check if count is to small
  Edge : Inport
  Reset : Inport  Port=2
  IncsPerTurn : Inport  Port=3
  Dir : Inport  Port=4
  Position_offset : Inport  Port=5
  Add1 : Sum  AccumDataTypeStr=int16  OutDataTypeStr=int16
  Constant1 : Constant  Value=0  OutDataTypeStr=int16  SampleTime=-1
  Constant2 : Constant  OutDataTypeStr=int16  SampleTime=-1
  Constant3 : Constant  Value=0  OutDataTypeStr=int16  SampleTime=-1
  Constant5 : Constant  Value=-1  OutDataTypeStr=int16  SampleTime=-1
  Relational Operator : RelationalOperator  Operator=>  OutDataTypeStr=boolean  InputSameDT=off
  Relational Operator1 : RelationalOperator  Operator=<=  OutDataTypeStr=boolean  InputSameDT=off
  Resett_switch1 : Switch  Criteria=u2 ~= 0  OutDataTypeStr=uint16  SaturateOnIntegerOverflow=off  InputSameDT=off
  Resett_switch2 : Switch  Criteria=u2 ~= 0  OutDataTypeStr=int16  SaturateOnIntegerOverflow=off  InputSameDT=off
  Resett_switch3 : Switch  Criteria=u2 ~= 0  OutDataTypeStr=int16  SaturateOnIntegerOverflow=off  InputSameDT=off
  Subsystem : Subsystem  Commented=on
  only_use_for_neg_speed : Switch  Threshold=1  SaturateOnIntegerOverflow=off  InputSameDT=off
  reset_old{1..7} (7 alike) : Delay  DelayLength=1
  speed_old_switch1 : Switch  Criteria=u2 ~= 0  SaturateOnIntegerOverflow=off  InputSameDT=off
  speed_old_switch2 : Switch  Threshold=1  SaturateOnIntegerOverflow=off  InputSameDT=off
  count : Outport  VectorParamsAs1DForOutWhenUnconnected=off
  wires:
  reset_old7/1 -> Resett_switch2/1
  reset_old6/1 -> speed_old_switch2/2, only_use_for_neg_speed/2
  Dir/1 -> reset_old6/1
  Add1/1 -> Resett_switch2/3
  Position_offset/1 -> reset_old7/1
  reset_old1/1 -> Add1/2
  Edge/1 -> speed_old_switch1/2
  reset_old2/1 -> only_use_for_neg_speed/3
  Reset/1 -> Resett_switch2/2
  IncsPerTurn/1 -> reset_old5/1
  Constant3/1 -> speed_old_switch1/3
  Constant1/1 -> Resett_switch1/1, Relational Operator1/2, only_use_for_neg_speed/1
  Resett_switch1/1 -> reset_old1/1, count/1, Relational Operator/1
  reset_old3/1 -> Resett_switch1/2
  Relational Operator1/1 -> reset_old2/1
  speed_old_switch2/1 -> reset_old4/1
  Resett_switch3/1 -> Resett_switch1/3, Relational Operator1/1
  only_use_for_neg_speed/1 -> Resett_switch3/2
  Resett_switch2/1 -> Resett_switch3/3
  reset_old5/1 -> Relational Operator/2, Resett_switch3/1
  reset_old4/1 -> speed_old_switch1/1
  Constant2/1 -> speed_old_switch2/1
  Relational Operator/1 -> reset_old3/1
  Constant5/1 -> speed_old_switch2/3
  speed_old_switch1/1 -> Add1/1

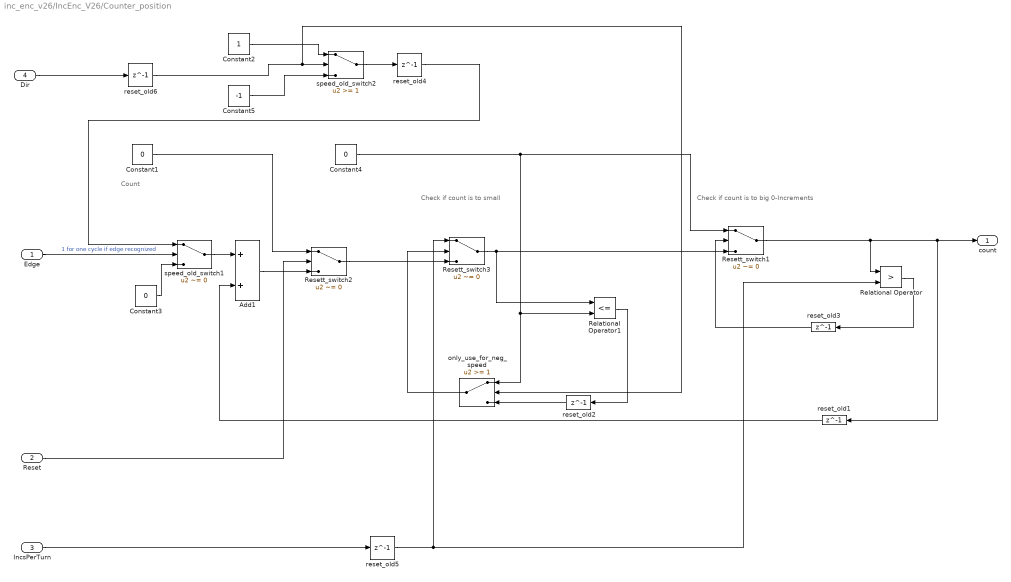
== system inc_enc_v26/IncEnc_V26/Counter_position ==
  note: Count
  note: Check if count is to big 0-Increments
  note: Check if count is to small
  Edge : Inport
  Reset : Inport  Port=2
  IncsPerTurn : Inport  Port=3
  Dir : Inport  Port=4
  Add1 : Sum  AccumDataTypeStr=int16  OutDataTypeStr=int16
  Constant1 : Constant  Value=0  OutDataTypeStr=int16  SampleTime=-1
  Constant2 : Constant  OutDataTypeStr=int16  SampleTime=-1
  Constant3 : Constant  Value=0  OutDataTypeStr=int16  SampleTime=-1
  Constant4 : Constant  Value=0  OutDataTypeStr=int16  SampleTime=-1
  Constant5 : Constant  Value=-1  OutDataTypeStr=int16  SampleTime=-1
  Relational Operator : RelationalOperator  Operator=>  OutDataTypeStr=boolean  InputSameDT=off
  Relational Operator1 : RelationalOperator  Operator=<=  OutDataTypeStr=boolean  InputSameDT=off
  Resett_switch1 : Switch  Criteria=u2 ~= 0  OutDataTypeStr=uint16  SaturateOnIntegerOverflow=off  InputSameDT=off
  Resett_switch2 : Switch  Criteria=u2 ~= 0  OutDataTypeStr=int16  SaturateOnIntegerOverflow=off  InputSameDT=off
  Resett_switch3 : Switch  Criteria=u2 ~= 0  OutDataTypeStr=int16  SaturateOnIntegerOverflow=off  InputSameDT=off
  only_use_for_neg_speed : Switch  Threshold=1  SaturateOnIntegerOverflow=off  InputSameDT=off
  reset_old{1..6} (6 alike) : Delay  DelayLength=1
  speed_old_switch1 : Switch  Criteria=u2 ~= 0  SaturateOnIntegerOverflow=off  InputSameDT=off
  speed_old_switch2 : Switch  Threshold=1  SaturateOnIntegerOverflow=off  InputSameDT=off
  count : Outport  VectorParamsAs1DForOutWhenUnconnected=off
  wires:
  Reset/1 -> Resett_switch2/2
  Edge/1 -> speed_old_switch1/2  "1 for one cycle if edge recognized"
  Add1/1 -> Resett_switch2/3
  speed_old_switch1/1 -> Add1/1
  Constant3/1 -> speed_old_switch1/3
  Constant2/1 -> speed_old_switch2/1
  Dir/1 -> reset_old6/1
  Constant5/1 -> speed_old_switch2/3
  speed_old_switch2/1 -> reset_old4/1
  Relational Operator/1 -> reset_old3/1
  Constant4/1 -> only_use_for_neg_speed/1, Relational Operator1/2, Resett_switch1/1
  Resett_switch2/1 -> Resett_switch3/3
  Resett_switch3/1 -> Relational Operator1/1, Resett_switch1/3
  Relational Operator1/1 -> reset_old2/1
  only_use_for_neg_speed/1 -> Resett_switch3/2
  reset_old4/1 -> speed_old_switch1/1
  IncsPerTurn/1 -> reset_old5/1
  reset_old6/1 -> only_use_for_neg_speed/2, speed_old_switch2/2
  Resett_switch1/1 -> Relational Operator/1, reset_old1/1, count/1
  reset_old3/1 -> Resett_switch1/2
  reset_old2/1 -> only_use_for_neg_speed/3
  reset_old5/1 -> Relational Operator/2, Resett_switch3/1
  reset_old1/1 -> Add1/2
  Constant1/1 -> Resett_switch2/1

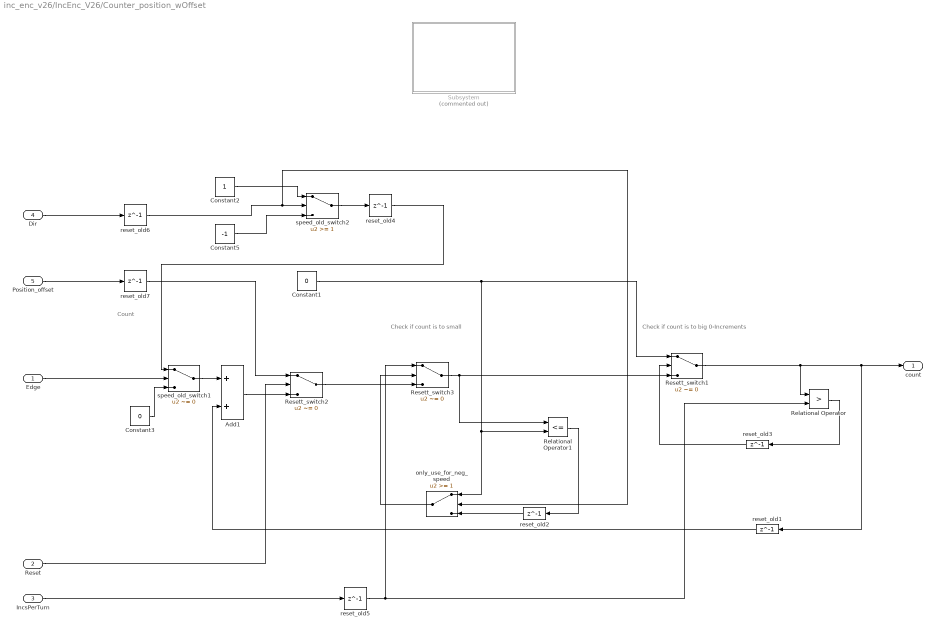
== system inc_enc_v26/IncEnc_V26/Counter_position_wOffset ==
  note: Check if count is to small
  note: Count
  note: Check if count is to big 0-Increments
  Edge : Inport
  Reset : Inport  Port=2
  IncsPerTurn : Inport  Port=3
  Dir : Inport  Port=4
  Position_offset : Inport  Port=5
  Add1 : Sum  AccumDataTypeStr=int16  OutDataTypeStr=int16
  Constant1 : Constant  Value=0  OutDataTypeStr=int16  SampleTime=-1
  Constant2 : Constant  OutDataTypeStr=int16  SampleTime=-1
  Constant3 : Constant  Value=0  OutDataTypeStr=int16  SampleTime=-1
  Constant5 : Constant  Value=-1  OutDataTypeStr=int16  SampleTime=-1
  Relational Operator : RelationalOperator  Operator=>  OutDataTypeStr=boolean  InputSameDT=off
  Relational Operator1 : RelationalOperator  Operator=<=  OutDataTypeStr=boolean  InputSameDT=off
  Resett_switch1 : Switch  Criteria=u2 ~= 0  OutDataTypeStr=uint16  SaturateOnIntegerOverflow=off  InputSameDT=off
  Resett_switch2 : Switch  Criteria=u2 ~= 0  OutDataTypeStr=int16  SaturateOnIntegerOverflow=off  InputSameDT=off
  Resett_switch3 : Switch  Criteria=u2 ~= 0  OutDataTypeStr=int16  SaturateOnIntegerOverflow=off  InputSameDT=off
  Subsystem : Subsystem  Commented=on
  only_use_for_neg_speed : Switch  Threshold=1  SaturateOnIntegerOverflow=off  InputSameDT=off
  reset_old{1..7} (7 alike) : Delay  DelayLength=1
  speed_old_switch1 : Switch  Criteria=u2 ~= 0  SaturateOnIntegerOverflow=off  InputSameDT=off
  speed_old_switch2 : Switch  Threshold=1  SaturateOnIntegerOverflow=off  InputSameDT=off
  count : Outport  VectorParamsAs1DForOutWhenUnconnected=off
  wires:
  speed_old_switch1/1 -> Add1/1
  Constant5/1 -> speed_old_switch2/3
  Relational Operator/1 -> reset_old3/1
  Constant2/1 -> speed_old_switch2/1
  reset_old4/1 -> speed_old_switch1/1
  reset_old5/1 -> Resett_switch3/1, Relational Operator/2
  Resett_switch2/1 -> Resett_switch3/3
  only_use_for_neg_speed/1 -> Resett_switch3/2
  Resett_switch3/1 -> Relational Operator1/1, Resett_switch1/3
  speed_old_switch2/1 -> reset_old4/1
  Relational Operator1/1 -> reset_old2/1
  reset_old3/1 -> Resett_switch1/2
  Resett_switch1/1 -> Relational Operator/1, count/1, reset_old1/1
  Constant1/1 -> only_use_for_neg_speed/1, Relational Operator1/2, Resett_switch1/1
  Constant3/1 -> speed_old_switch1/3
  IncsPerTurn/1 -> reset_old5/1
  Reset/1 -> Resett_switch2/2
  reset_old2/1 -> only_use_for_neg_speed/3
  Edge/1 -> speed_old_switch1/2
  reset_old1/1 -> Add1/2
  Position_offset/1 -> reset_old7/1
  Add1/1 -> Resett_switch2/3
  Dir/1 -> reset_old6/1
  reset_old6/1 -> only_use_for_neg_speed/2, speed_old_switch2/2
  reset_old7/1 -> Resett_switch2/1

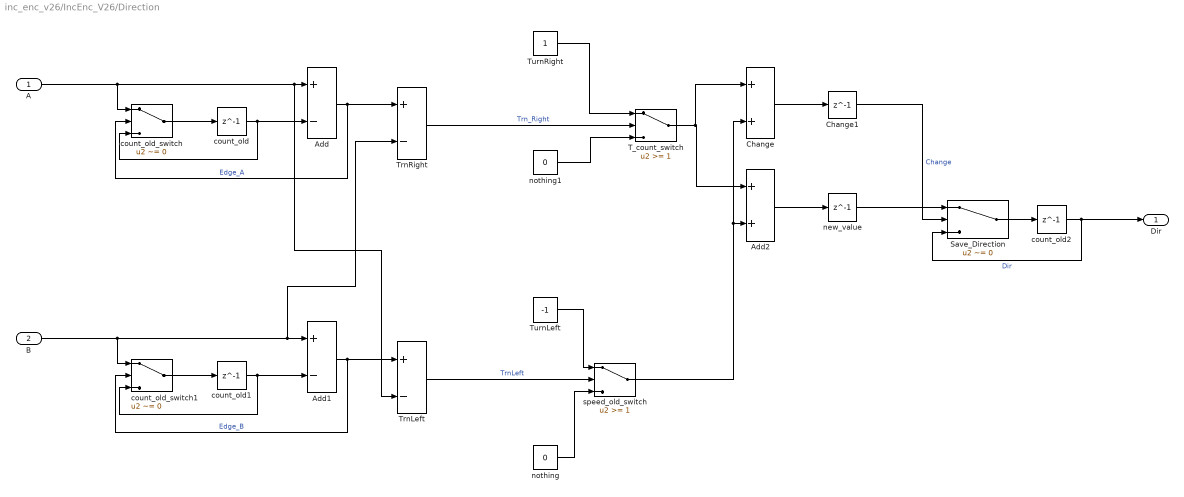
== system inc_enc_v26/IncEnc_V26/Direction ==
  A : Inport
  B : Inport  Port=2
  Add : Sum  Inputs=+-  AccumDataTypeStr=fixdt(1,4,0)  OutDataTypeStr=fixdt(1,4,0)
  Add1 : Sum  Inputs=+-  AccumDataTypeStr=fixdt(1,4,0)  OutDataTypeStr=fixdt(1,4,0)
  Add2 : Sum  AccumDataTypeStr=fixdt(1,4,0)  OutDataTypeStr=fixdt(1,4,0)
  Change : Sum  AccumDataTypeStr=fixdt(1,4,0)  OutDataTypeStr=fixdt(1,4,0)
  Change1 : Delay  DelayLength=1
  Save_Direction : Switch  Criteria=u2 ~= 0  Threshold=0.1  OutDataTypeStr=fixdt(1,4,0)  SaturateOnIntegerOverflow=off  InputSameDT=off
  T_count_switch : Switch  Threshold=1  OutDataTypeStr=Inherit: Inherit via back propagation  SaturateOnIntegerOverflow=off  InputSameDT=off
  TrnLeft : Sum  Inputs=+-  AccumDataTypeStr=fixdt(1,4,0)  OutDataTypeStr=fixdt(1,4,0)
  TrnRight : Sum  Inputs=+-  AccumDataTypeStr=fixdt(1,4,0)  OutDataTypeStr=fixdt(1,4,0)
  TurnLeft : Constant  Value=-1  OutDataTypeStr=fixdt(1,4,0)  SampleTime=-1
  TurnRight : Constant  OutDataTypeStr=fixdt(1,4,0)  SampleTime=-1
  count_old : Delay  DelayLength=1
  count_old1 : Delay  DelayLength=1
  count_old2 : Delay  DelayLength=1
  count_old_switch : Switch  Criteria=u2 ~= 0  OutDataTypeStr=Inherit: Inherit via back propagation  SaturateOnIntegerOverflow=off  InputSameDT=off
  count_old_switch1 : Switch  Criteria=u2 ~= 0  OutDataTypeStr=Inherit: Inherit via back propagation  SaturateOnIntegerOverflow=off  InputSameDT=off
  new_value : Delay  DelayLength=1
  nothing : Constant  Value=0  OutDataTypeStr=fixdt(1,4,0)  SampleTime=-1
  nothing1 : Constant  Value=0  OutDataTypeStr=fixdt(1,4,0)  SampleTime=-1
  speed_old_switch : Switch  Threshold=1  OutDataTypeStr=Inherit: Inherit via back propagation  SaturateOnIntegerOverflow=off  InputSameDT=off
  Dir : Outport  VectorParamsAs1DForOutWhenUnconnected=off
  wires:
  A/1 -> TrnLeft/2, Add/1, count_old_switch/1
  count_old_switch/1 -> count_old/1
  count_old/1 -> count_old_switch/3, Add/2
  TurnRight/1 -> T_count_switch/1
  Add/1 -> TrnRight/1, count_old_switch/2  "Edge_A"
  T_count_switch/1 -> Change/1, Add2/1
  Save_Direction/1 -> count_old2/1
  B/1 -> TrnRight/2, Add1/1, count_old_switch1/1
  count_old_switch1/1 -> count_old1/1
  count_old1/1 -> count_old_switch1/3, Add1/2
  Add1/1 -> TrnLeft/1, count_old_switch1/2  "Edge_B"
  TrnRight/1 -> T_count_switch/2  "Trn_Right"
  new_value/1 -> Save_Direction/1
  TrnLeft/1 -> speed_old_switch/2  "TrnLeft"
  TurnLeft/1 -> speed_old_switch/1
  nothing/1 -> speed_old_switch/3
  nothing1/1 -> T_count_switch/3
  speed_old_switch/1 -> Change/2, Add2/2
  Add2/1 -> new_value/1
  Change/1 -> Change1/1
  Change1/1 -> Save_Direction/2  "Change"
  count_old2/1 -> Save_Direction/3, Dir/1  "Dir"

== system inc_enc_v26/IncEnc_V26/Index_Latch ==
  Reset_in : Inport
  Constant : Constant  OutDataTypeStr=boolean  SampleTime=T_fpga
  Constant4 : Constant  Value=0  OutDataTypeStr=boolean  SampleTime=T_fpga
  Delay : Delay  DelayLength=1
  OR : Logic  Operator=OR  AllPortsSameDT=off  OutDataTypeStr=boolean
  Switch : Switch  Criteria=u2 > Threshold  SaturateOnIntegerOverflow=off  InputSameDT=off
  Index_found : Outport
  wires:
  Constant4/1 -> Switch/3
  Delay/1 -> OR/2
  Constant/1 -> Switch/1
  Switch/1 -> Index_found/1, Delay/1
  Reset_in/1 -> OR/1
  OR/1 -> Switch/2

== system inc_enc_v26/IncEnc_V26/count_lines ==
  note: Set new counter value
  note: Check if count is to big in order to safe for value overflow
  note: Count
  note: omega by counting lines, can be used for high-speed, but is not recommended for small drives!
      | However, for using this approach, we need a quite long time window in order to get an accurate speed.
      | For small drives a long time window is not acceptable, since the mechanical time constant is small.
      | e.g. using just 100us (since the speed control has this period at 10kHz) we can calculate as following:
      | speed = 5034rpm, Increments = 5000, QuadratureFactor = 4, f_cc = 10000 kHz
      | In the test, 169 lines are counted in 100us in the described example.
      | -> 169*(10000/(4*5000))*60 = 5070rpm (so this is not accurate!)
      | However, a longer time window is not acceptabel for speed control with10kHz. More increments is not common, since 5000 are already a lot!
  Edge : Inport
  Reset : Inport  Port=2
  IncsPerTurn : Inport  Port=3
  Add1 : Sum  AccumDataTypeStr=int16  OutDataTypeStr=int16
  Constant1 : Constant  Value=0  OutDataTypeStr=int16  SampleTime=-1
  Constant2 : Constant  OutDataTypeStr=int16  SampleTime=-1
  Constant3 : Constant  Value=0  OutDataTypeStr=int16  SampleTime=-1
  Constant4 : Constant  Value=10  OutDataTypeStr=int16  SampleTime=-1
  Relational Operator : RelationalOperator  Operator=>  OutDataTypeStr=boolean  InputSameDT=off
  Reset_when_overflow : Sum  OutDataTypeStr=int16
  Resett_switch1 : Switch  Criteria=u2 ~= 0  OutDataTypeStr=int16  SaturateOnIntegerOverflow=off  InputSameDT=off
  Resett_switch2 : Switch  Criteria=u2 ~= 0  OutDataTypeStr=int16  SaturateOnIntegerOverflow=off  InputSameDT=off
  reset_old{1,3..5} (4 alike) : Delay  DelayLength=1
  reset_old_switch1 : Switch  Criteria=u2 ~= 0  SaturateOnIntegerOverflow=off  InputSameDT=off
  speed_old_switch1 : Switch  Criteria=u2 ~= 0  SaturateOnIntegerOverflow=off  InputSameDT=off
  count : Outport  VectorParamsAs1DForOutWhenUnconnected=off
  wires:
  Reset_when_overflow/1 -> reset_old5/1
  Relational Operator/1 -> Resett_switch1/2
  speed_old_switch1/1 -> Add1/1
  reset_old5/1 -> Relational Operator/2
  Resett_switch2/1 -> Resett_switch1/3
  reset_old4/1 -> speed_old_switch1/1
  Edge/1 -> speed_old_switch1/2  "1 for one cycle if edge recognized"
  Constant1/1 -> Resett_switch2/1, Resett_switch1/1
  Constant3/1 -> speed_old_switch1/3
  IncsPerTurn/1 -> Reset_when_overflow/2
  Add1/1 -> Resett_switch2/3
  Constant2/1 -> reset_old4/1
  Constant4/1 -> Reset_when_overflow/1
  Resett_switch1/1 -> reset_old3/1
  reset_old3/1 -> reset_old_switch1/1, Add1/2, Relational Operator/1
  reset_old1/1 -> reset_old_switch1/3
  Reset/1 -> reset_old_switch1/2, Resett_switch2/2  "Use new value"
  reset_old_switch1/1 -> reset_old1/1, count/1

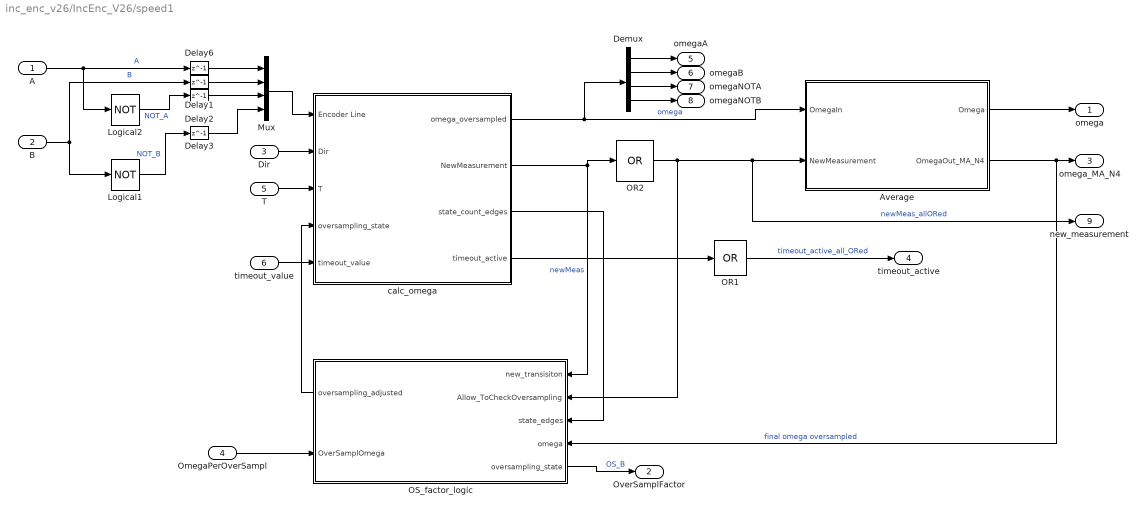
== system inc_enc_v26/IncEnc_V26/speed1 ==
  A : Inport
  B : Inport  Port=2
  Dir : Inport  Port=3
  OmegaPerOverSampl : Inport  Port=4
  T : Inport  Port=5
  timeout_value : Inport  Port=6  OutDataTypeStr=uint32
  Average : Subsystem
  Delay{1..3,6} (4 alike) : Delay  DelayLength=1  InitialCondition=0
  Demux : Demux
  Logical1 : Logic  Operator=NOT  AllPortsSameDT=off  OutDataTypeStr=boolean
  Logical2 : Logic  Operator=NOT  AllPortsSameDT=off  OutDataTypeStr=boolean
  Mux : Mux
  OR1 : Logic  Operator=OR  Inputs=1  AllPortsSameDT=off  OutDataTypeStr=boolean
  OR2 : Logic  Operator=OR  Inputs=1  AllPortsSameDT=off  OutDataTypeStr=boolean
  OS_factor_logic : Subsystem
      settings: PortSchema="{\"entries\":[{\"content\":{\"sides\":[{\"content\":{\"connectorIds\":[\"In1\",\"In2\",\"In3\",\"In4\",\"Out2\"]},\"type\":\"ConnectorPlacement.EquallySpacedRectSide\",\"uuid\":\"00190a63-1990-4dc8-8561-af6346041cd2\"},{\"content\":{\"connectorIds\":[\"Out1\",\"In5\"],\"side\":\"RIGHT\"},\"type\":\"ConnectorPlacement.EquallySpacedRectSide\",\"uuid\":\"ed8fa1bb-ba76-4f60-9676-d72d7f094a86\"},{\"content\":{\"connectorIds\":[],\"side\":\"TOP\"},\"type\":\"ConnectorPlacement.EquallySpacedRectSide\",\"uuid\":\"16aa4cab-6298-4523-a92b-d078d21511a0\"}]},\"type\":\"ConnectorPlacement.EquallySpacedConnector\",\"uuid\":\"bb0c721d-662f-49b4-b1e3-cc7ff0334cdb\"}],\"packageUris\":[\"http://schema.mathworks.com/mf0/Connector/R2020b\"],\"version\":\"1.0\"}"
  calc_omega : Subsystem  TreatAsAtomicUnit=on
  omega : Outport  VectorParamsAs1DForOutWhenUnconnected=off
  OverSamplFactor : Outport  Port=2
  omega_MA_N4 : Outport  Port=3  VectorParamsAs1DForOutWhenUnconnected=off
  timeout_active : Outport  Port=4  OutDataTypeStr=boolean  VectorParamsAs1DForOutWhenUnconnected=off
  omegaA : Outport  Port=5  VectorParamsAs1DForOutWhenUnconnected=off
  omegaB : Outport  Port=6  VectorParamsAs1DForOutWhenUnconnected=off
  omegaNOTA : Outport  Port=7  VectorParamsAs1DForOutWhenUnconnected=off
  omegaNOTB : Outport  Port=8  VectorParamsAs1DForOutWhenUnconnected=off
  new_measurement : Outport  Port=9  OutDataTypeStr=boolean  VectorParamsAs1DForOutWhenUnconnected=off
  wires:
  Dir/1 -> calc_omega/2(Dir)
  B/1 -> Delay1/1, Logical1/1  "B"
  OmegaPerOverSampl/1 -> OS_factor_logic/5(OverSamplOmega)
  OR2/1 -> OS_factor_logic/2(Allow_ToCheckOversampling), Average/2(NewMeasurement), new_measurement/1  "newMeas_allORed"
  OS_factor_logic/2(oversampling_state) -> OverSamplFactor/1  "OS_B"
  OR1/1 -> timeout_active/1  "timeout_active_all_ORed"
  Average/2(OmegaOut_MA_N4) -> omega_MA_N4/1, OS_factor_logic/4(omega)  "final omega oversampled"
  A/1 -> Logical2/1, Delay6/1  "A"
  Mux/1 -> calc_omega/1(Encoder Line)
  T/1 -> calc_omega/3(T)
  timeout_value/1 -> calc_omega/5(timeout_value)
  Demux/2 -> omegaB/1
  Demux/1 -> omegaA/1
  Demux/4 -> omegaNOTB/1
  Demux/3 -> omegaNOTA/1
  calc_omega/1(omega_oversampled) -> Demux/1, Average/1("OmegaIn ")  "omega"
  calc_omega/2(NewMeasurement) -> OR2/1, OS_factor_logic/1(new_transisiton)  "newMeas"
  calc_omega/3(state_count_edges) -> OS_factor_logic/3(state_edges)
  calc_omega/4(timeout_active) -> OR1/1
  Logical2/1 -> Delay2/1  "NOT_A"
  Logical1/1 -> Delay3/1  "NOT_B"
  OS_factor_logic/1(oversampling_adjusted) -> calc_omega/4(oversampling_state)
  Delay6/1 -> Mux/1
  Delay1/1 -> Mux/2
  Delay2/1 -> Mux/3
  Delay3/1 -> Mux/4
  Average/1(Omega) -> omega/1
